simulink model "VEHICLE_DYN_TRAIN"  (R2019b)
settings: Solver=ode4  StartTime=0.0  StopTime=150  FixedStep=0.01  RelTol=1e-3
model workspace (MAT data in the model file):
  ACCEL = [0 0.000975932898663 -0.0414538855996 0.0440661905922 -0.0484817487001 0.0392964510644 -0.0693895143615 0.0261566921783 -0.0586295561215 0.0249771458914 -0.0595081132089 0.0233316013131 ... (544 elements, 17x32)]
  A_mc = 0.000491
  CMD_BR = [0 0 0 0 0 0 0 0 0 0 0 0 ... (15001 elements, 15001x1)]
  CMD_MODE = [1 1 1 1 1 1 1 1 1 1 1 1 ... (15001 elements, 15001x1)]
  CMD_ST = [0 0 0 0 0 0 0 0 0 0 0 0 ... (15001 elements, 15001x1)]
  CMD_T = [0 0.01 0.02 0.03 0.04 0.05 0.06 0.07 0.08 0.09 0.1 0.11 ... (2001 elements, 1x2001)]
  CMD_TH = [0 0 0 0 0 0 0 0 0 0 0 0 ... (15001 elements, 15001x1)]
  CMD_TM = [0 0.01 0.02 0.03 0.04 0.05 0.06 0.07 0.08 0.09 0.1 0.11 ... (15001 elements, 15001x1)]
  CMD_U = [10 10 10 10 10 10 10 10 10 10 10 10 ... (2001 elements, 1x2001)]
  CMD_UX = [0.1 0.1 0.1 0.1 0.1 0.1 0.1 0.1 0.1 0.1 0.1 0.1 ... (15001 elements, 15001x1)]
  COMMAND = [0  0  0  0  0  0; 0  0  0  0  -183.19381415  -6.40437742372; 0  0  0  0  1801.61134482  -6.40437742372; 0  0  0  0  -3911.54207947  -6.40437742372; 0  0  0  0  5117.32624779  -6.40437742372; 0  0  0  0  -8382.76633117  -6.40437742372; 0  0  0  0  5855.89111168  -6.40437742372; 0  0  0  0  2797.21692809  -6.40437742372; 0  0  0  0  -3762.9671569  -6.40437742372; 0  0  0  0  4210.58821039  -6.40437742372; 0  0  0  0  -2996.08013613  -6.40437742372; 0  0  0  0  5501.10926406  -6.40437742372; 0  0  0  0  1163.55068011  -6.40437742372; 0  0  0  0  -217.743214556  -6.40437742372; 0  0  0  0  2898.65655248  -6.40437742372; 0  0  0  0  2351.72581017  -6.40437742372; 0  0  0  0  936.262311224  -6.40437742372]
  C_q = 1.4e-06
  DATA_HMMWV.g = 9.81
  DATA_HMMWV.MU = 109.293567034
  DATA_HMMWV.MS = 2251.54374814
  DATA_HMMWV.VEHICLEMASS = 2688.71801627
  DATA_HMMWV.LA = 1.577476562
  DATA_HMMWV.LB = 1.724523438
  DATA_HMMWV.LC = 1.819402
  DATA_HMMWV.IXX = 1186.25695083
  DATA_HMMWV.IYY = 3535.89110102
  DATA_HMMWV.IZZ = 4110.07986387
  DATA_HMMWV.KS = [56433.9261732 56433.9261732 102219.884388 102219.884388]
  DATA_HMMWV.KT = [784944 784944 784944 784944]
  DATA_HMMWV.CS.RS = [-0.3391408 -0.332289470707 -0.325438141414 -0.318586812121 -0.311735482828 -0.304884153535 -0.298032824242 -0.291181494949 -0.284330165657 -0.277478836364 -0.270627507071 -0.263776177778 -0.256924848485 -0.250073519192 -0.243222189899 -0.236370860606 -0.229519531313 -0.22266820202 -0.215816872727 -0.208965543434 -0.202114214141 -0.195262884848 -0.188411555556 -0.181560226263 -0.17470889697 -0.167857567677 -0.161006238384 -0.154154909091 -0.147303579798 -0.140452250505 -0.133600921212 -0.126749591919 -0.119898262626 -0.113046933333 -0.10619560404 -0.0993442747475 -0.0924929454545 -0.0856416161616 -0.0787902868687 -0.0719389575758 -0.0650876282828 -0.0582362989899 -0.051384969697 -0.044533640404 -0.0376823111111 -0.0308309818182 -0.0239796525253 -0.0171283232323 -0.0102769939394 -0.00342566464646 0.00342566464646 0.0102769939394 0.0171283232323 0.0239796525253 0.0308309818182 0.0376823111111 0.044533640404 0.051384969697 0.0582362989899 0.0650876282828 0.0719389575758 0.0787902868687 0.0856416161616 0.0924929454545 0.0993442747475 0.10619560404 0.113046933333 0.119898262626 0.126749591919 0.133600921212 0.140452250505 0.147303579798 0.154154909091 0.161006238384 0.167857567677 0.17470889697 0.181560226263 0.188411555556 0.195262884848 0.202114214141 0.208965543434 0.215816872727 0.22266820202 0.229519531313 0.236370860606 0.243222189899 0.250073519192 0.256924848485 0.263776177778 0.270627507071 0.277478836364 0.284330165657 0.291181494949 0.298032824242 0.304884153535 0.311735482828 0.318586812121 0.325438141414 0.332289470707 0.3391408]
  DATA_HMMWV.CS.FDF = [-4248.0516471 -4239.67420418 -4225.63626971 -4206.16859138 -4181.50191691 -4151.866994 -4117.49457036 -4078.6153937 -4035.46021171 -3988.25977212 -3937.24482263 -3882.64611094 -3824.69438476 -3763.62039179 -3699.65487975 -3633.02859634 -3563.97228926 -3492.71670623 -3419.49259495 -3344.53070313 -3268.06177847 -3190.31656868 -3111.52582147 -3031.92028454 -2951.7307056 -2870.62252603 -2776.89068437 -2667.42140814 -2544.36901672 -2409.88782945 -2266.13216571 -2115.25634485 -1959.41468624 -1800.76150924 -1641.4511332 -1483.63787749 -1329.47606146 -1181.12000449 -1040.72402593 -910.442445139 -792.429581481 -688.738492968 -597.716409788 -515.80816219 -440.03739839 -367.427766603 -295.002915045 -219.786491931 -138.802145476 -49.0735238952 51.8288236509 162.22936071 281.055193785 407.628054481 541.269674406 681.301785165 827.046118366 977.824405614 1132.95837852 1295.36858067 1472.0381359 1661.32419521 1861.23445035 2069.77659305 2284.95831505 2504.78730808 2727.27126389 2950.4178742 3172.23483076 3390.7298253 3603.91054956 3809.78469528 4006.35995418 4191.64401802 4363.64457851 4524.5756402 4683.55471804 4840.88541831 4996.44105067 5150.09492481 5301.72035039 5451.1906371 5598.3790946 5743.15903257 5885.40376068 6024.98658862 6161.78082604 6295.65978264 6426.49676807 6554.16509202 6678.53806417 6799.48899417 6916.89119172 7030.61796648 7140.54262813 7246.53848634 7348.47885079 7446.23703115 7539.68633709 7628.7000783]
  DATA_HMMWV.CS.FDR = [-4359.2571876 -4354.21629512 -4343.74283127 -4328.06230688 -4307.40023276 -4281.98211973 -4252.03347861 -4217.7798202 -4179.44665534 -4137.25949483 -4091.4438495 -4042.22523015 -3989.82914761 -3934.4811127 -3876.40663622 -3815.831229 -3752.98040185 -3688.07966559 -3621.35453104 -3553.030509 -3483.33311031 -3412.48784578 -3340.72022622 -3268.25576245 -3195.31996528 -3121.7277695 -3038.93655817 -2944.39727451 -2839.35128227 -2725.03994522 -2602.70462711 -2473.58669171 -2338.92750277 -2199.96842406 -2057.95081932 -1914.11605233 -1769.70548684 -1625.96048661 -1484.1224154 -1345.43263697 -1211.13251508 -1082.42805518 -958.881518595 -838.498018865 -719.350253999 -599.510922001 -477.052720875 -350.048348627 -216.570503261 -74.6918827812 77.318355522 239.265853953 410.47181173 590.349120247 778.3106709 973.769355084 1176.13806419 1384.82968962 1599.25712277 1821.34171769 2055.89543661 2301.77114007 2557.5791448 2821.92976751 3093.43332495 3370.70013382 3652.34051085 3936.96477277 4223.18323631 4509.60621818 4794.8440351 5077.50700382 5356.20544104 5629.5496635 5896.14998792 6156.94821393 6416.88709644 6676.18645946 6934.83106248 7192.80566502 7450.09502655 7706.68390659 7962.55706462 8217.69926015 8472.09525268 8725.7298017 8978.58766672 9230.65360722 9481.91238271 9732.34875269 9981.94747665 10230.6933141 10478.5710245 10725.5653674 10971.6611023 11216.8429887 11461.095786 11704.4042538 11946.7531516 12188.1272388]
  DATA_HMMWV.CS.RS_INIT = -0.3391408
  DATA_HMMWV.CS.RS_SLOPE = 145.957077414
  DATA_HMMWV.AREA_FRONTAL = 3.58
  DATA_HMMWV.AIR_DENSITY = 1.22
  DATA_HMMWV.DRAG_COEFF = 0.7
  DATA_HMMWV.MAXPOWER = 225000
  DATA_HMMWV.IW = [40 40 40 40]
  DATA_HMMWV.RW = [0.548 0.548 0.548 0.548]
  DATA_HMMWV.HRCF = 0.85
  DATA_HMMWV.HRCR = 0.9
  DATA_HMMWV.HG = 0.9902452
  DATA_HMMWV.ZS_INIT = [0.9902452 0.9902452 0.9902452 0.9902452]
  DATA_HMMWV.XS_INIT = [-0.102204770695 -0.102204770695 -0.0516142786918 -0.0516142786918]
  DATA_HMMWV.XT_INIT = [-0.0087748080939 -0.0087748080939 -0.00802659668124 -0.00802659668124]
  DATA_HMMWV.ZT_INIT = [0.539225191906 0.539225191906 0.539973403319 0.539973403319]
  DATA_VESIM_CC_BRAKE.A_mc = 0.000491
  DATA_VESIM_CC_BRAKE.C_q = 1.4e-06
  DATA_VESIM_CC_BRAKE.F_cf = 80
  DATA_VESIM_CC_BRAKE.F_cs = 138
  DATA_VESIM_CC_BRAKE.F_z = -50097.6
  DATA_VESIM_CC_BRAKE.Gain_v = 70
  DATA_VESIM_CC_BRAKE.J_wheel = 32
  DATA_VESIM_CC_BRAKE.K_vb = 1500
  DATA_VESIM_CC_BRAKE.Kp_rpm = 2.7013
  DATA_VESIM_CC_BRAKE.Kp_v = 30
  DATA_VESIM_CC_BRAKE.L3 = 10
  DATA_VESIM_CC_BRAKE.MIN_TH = 0
  DATA_VESIM_CC_BRAKE.M_sprung = 4672
  DATA_VESIM_CC_BRAKE.M_unsprung = 220
  DATA_VESIM_CC_BRAKE.M_unsprung_front = 220
  DATA_VESIM_CC_BRAKE.M_vehicle = 5112
  DATA_VESIM_CC_BRAKE.N2 = 0
  DATA_VESIM_CC_BRAKE.N3 = 0.01
  DATA_VESIM_CC_BRAKE.P = 36
  DATA_VESIM_CC_BRAKE.P_0 = 10670
  DATA_VESIM_CC_BRAKE.P_gain = 0.0006
  DATA_VESIM_CC_BRAKE.R_wheel = 0.4412
  DATA_VESIM_CC_BRAKE.S_o = 3
  DATA_VESIM_CC_BRAKE.T2_r = 4
  DATA_VESIM_CC_BRAKE.Ti_rpm = 0.6464
  DATA_VESIM_CC_BRAKE.Ti_v = 2.5
  DATA_VESIM_CC_BRAKE.Tt_rpm = 0.0808
  DATA_VESIM_CC_BRAKE.Tt_v = 0.3125
  DATA_VESIM_CC_BRAKE.b = 170
  DATA_VESIM_CC_BRAKE.brake_Pw = [-3.96235801772; -3.96238075942; -0.895107722214; -0.895547395081; 35.9159438465; 72.7273668629; 152.485661058; 244.514654481; 330.408495385; 364.152342142; 462.316700341; 535.939857177; 618.766076338; 698.524620692; 775.215566044; 873.379969726; 950.0709454; 1029.82956556; 1106.52050333; 1174.00856829; 1241.49660293; 1339.66109; 1401.01384325; 1486.90776754; 1535.98996559; 1600.4103709; 1664.83081412; 1704.7101242; 1741.52177464; 1784.46875952; 1812.07749166; 1879.56559453; 1910.24195599; 1968.52709508; 2042.15044143; 2097.36794361; 2155.65309786; 2223.14114766; 2281.42629432; 2342.77908548]
  DATA_VESIM_CC_BRAKE.brake_V = [-1.14468402636e-08; 6.09303685082e-09; 2.9257815427e-07; 6.31682445149e-07; 8.18779962309e-07; 1.05849711081e-06; 1.41515318379e-06; 1.67826507702e-06; 1.8361367918e-06; 2.02323385108e-06; 2.22788040303e-06; 2.46760304614e-06; 2.60793442592e-06; 2.77165185063e-06; 2.90028906324e-06; 3.06985586096e-06; 3.17510657075e-06; 3.28035773841e-06; 3.41484157672e-06; 3.50255103574e-06; 3.61364699758e-06; 3.71890091255e-06; 3.82414933291e-06; 3.91770816494e-06; 4.00541487665e-06; 4.10481712919e-06; 4.17498625321e-06; 4.22761183705e-06; 4.29193021441e-06; 4.32116975331e-06; 4.3737935056e-06; 4.4322698361e-06; 4.49658729769e-06; 4.57844875735e-06; 4.67200575784e-06; 4.74802013391e-06; 4.81818834217e-06; 4.91759105259e-06; 4.99360588655e-06; 5.06962117839e-06]
  DATA_VESIM_CC_BRAKE.diff_efficiency = 0.94
  DATA_VESIM_CC_BRAKE.diff_wRatio = 6.052
  DATA_VESIM_CC_BRAKE.diff_w_ratio = 3.56
  DATA_VESIM_CC_BRAKE.engine_inertia = 0.53
  DATA_VESIM_CC_BRAKE.fmin_mg = [42.75 43.31 51.6 64.3 73.65 71.1 72.7 72.36]
  DATA_VESIM_CC_BRAKE.fmin_mg_na = [42.79 42.79 42.79 42.79 42.79 42.79 42.79 42.79]
  DATA_VESIM_CC_BRAKE.g = -9.8
  DATA_VESIM_CC_BRAKE.g_motor_eff = 1
  DATA_VESIM_CC_BRAKE.gr_motor = 0
  DATA_VESIM_CC_BRAKE.mdot_fuel = [5e-06 1e-05 2e-05 3e-05 4e-05 5e-05 6e-05 7e-05 8e-05]
  DATA_VESIM_CC_BRAKE.ms2mph = 2.23694
  DATA_VESIM_CC_BRAKE.n_tire = 4
  DATA_VESIM_CC_BRAKE.no_cyl = 8
  DATA_VESIM_CC_BRAKE.rpm0 = 83.7758040957
  DATA_VESIM_CC_BRAKE.rpm0_c = 1000
  DATA_VESIM_CC_BRAKE.rpm2rads = 0.10471975512
  DATA_VESIM_CC_BRAKE.rpm_e = [50 800 1000 1500 2000 2500 3000 3300]
  DATA_VESIM_CC_BRAKE.rpm_engine = [700 800 1000 1500 2000 2500 3000 3300]
  DATA_VESIM_CC_BRAKE.rpm_hi_idle = 3400
  DATA_VESIM_CC_BRAKE.rpm_idle = 750
  DATA_VESIM_CC_BRAKE.rpm_max_c = 3200
  DATA_VESIM_CC_BRAKE.rpm_rated = 3200
  DATA_VESIM_CC_BRAKE.torque_engine = [9.767  75.383  190.94  285.59  359.33  412.18  444.11  455.15  465.28; 15.303  80.318  196.25  293.4  371.76  431.33  472.12  494.11  497.32; 12.411  76.501  195.96  303.79  399.98  484.55  557.5  618.81  668.49; -4.524  61.314  188.26  308.88  423.2  531.2  632.9  728.28  817.34; -12.214  53.908  182.37  305.8  424.19  537.55  645.86  749.14  847.39; -35.77  30.439  158.78  281.67  399.12  511.13  617.7  718.82  814.5; -70  0  142.48  247.52  352.56  457.6  562.64  667.68  772.72; -75.889  -0.746  128.13  228.45  321.9  435.11  548.32  661.53  774.74]
  DATA_VESIM_CC_BRAKE.trq_scale = 0.46
  FORCE = [0 -4628.45620853 2357.84853747 -1841.82564621 -1727.75397473 1695.19792057 -1263.06335256 1524.31841051 -1649.98396845 -1537.1025145 -1335.96213703 1639.88309903 ... (493 elements, 17x29)]
  F_cf = 80
  F_cs = 138
  F_z = -50097.6
  Gain_v = 70
  J_wheel = 32
  K_vb = 1500
  Kp_rpm = 2.7013
  Kp_v = 30
  L3 = 10
  MIN_TH = 0
  M_sprung = 4672
  M_unsprung = 220
  M_unsprung_front = 220
  M_vehicle = 5112
  N2 = 0
  N3 = 0.01
  P = 36
  P_0 = 10670
  P_gain = 0.0006
  R_wheel = 0.4412
  SLIP = [0  0  0  0  0  0  0  0; -0.5  -0.5  -0.5  -0.5  -0.0351887274111  -0.0353738230462  -0.0256932606875  -0.025828461899; 0.5  0.5  0.5  0.5  0.935278264578  0.935683083202  0.934894152193  0.935259838194; -0.5  -0.5  -0.5  -0.5  -1.13059878896  -1.14410835605  -1.11878156022  -1.13275622068; -0.5  -0.5  -0.5  -0.5  1.27459495579  1.23136771502  1.24805246322  1.20169616214; 0.5  0.5  0.5  0.5  -1.39209196917  -1.31492534486  -1.36213294459  -1.27313134121; -0.5  -0.5  -0.5  -0.5  1.53834230958  1.52444006435  1.53915754649  1.52553193263; 0.5  -0.5  0.5  0.5  -1.53769354144  -1.55669825468  -1.53887189115  -1.55713779288; -0.5  -0.5  -0.5  -0.5  1.20354096649  1.12996957728  1.14188288665  1.05975342846; -0.5  0.5  -0.5  -0.5  -1.39844393881  -1.41657840122  -1.39247530022  -1.41016962351; -0.5  0.5  0.5  0.5  1.45508387354  1.20457176324  1.49318511219  1.31789576983; 0.5  0.5  -0.5  -0.5  -1.43949280681  -1.45477228425  -1.43518373844  -1.45165922694; -0.5  -0.5  -0.5  -0.409071280156  1.31587025686  1.35042722118  1.33080027133  1.36372378815; 0.5  0.5  0.5  0.5  -1.49514740357  -1.52618133061  -1.49024093571  -1.52178551982; -0.5  -0.5  -0.5  -0.5  0.548035911605  0.535056729347  0.504680092205  0.492118930826; 0.5  0.5  0.5  0.5  -1.44242137448  -1.56048589042  -1.46811475456  -1.56157095897; 0.5  0.5  0.5  -0.5  1.45666931557  1.52468060226  1.41014141796  1.50590281378]
  STATE = [0 4.33747954961e-06 -0.000147430460781 -3.72129119222e-05 -0.000284189368187 -0.000207128204422 -0.00055150808757 -0.000594561033148 -0.000967775941564 -0.00103412952076 -0.00143215770154 -0.00152470872631 ... (544 elements, 17x32)]
  STATES_INIT = [0 0 0.9902452 0 0 1.57079632679 0.01 0 0 0 0 0 0 0 0 0 -0.0087748080939 -0.0087748080939 -0.00802659668124 -0.00802659668124 -0.102204770695 -0.102204770695 -0.0516142786918 -0.0516142786918 0.0185451276203 0.0185451276203 0.0185194306581 0.0185194306581 0 0 0 0]
  SUSP = [0 -0.00875795294893 -0.00878173856984 -0.00830852863719 -0.00873591176348 -0.00870428588158 -0.00751721170558 -0.00851904716693 -0.00789923296531 -0.00838039895253 -0.00756270047902 -0.00866403364289 ... (612 elements, 17x36)]
  S_o = 3
  T2_r = 4
  TIRE = [0 0.0910654620457 -0.0936729683319 0.0717372732987 0.0513932148365 -0.0365035701266 -0.00739813929507 -0.0045484168787 0.0723881675257 0.0296400174207 -0.0169805208571 0.0207214713062 ... (408 elements, 17x24)]
  TIRELIFTOFF = [0; 0; 0; 0; 0; 0; 0; 0; 0; 0; 0; 0; 0; 0; 0; 0; 0]
  T_LENGTH = 2001
  T_STEP = 0.01
  T_STOP = 12.82
  T_TOTAL = 20
  Ti_rpm = 0.6464
  Ti_v = 2.5
  Tstop = [150 150 150 150 150 150 150 150 150 150 150 150 ... (15001 elements, 15001x1)]
  Tt_rpm = 0.0808
  Tt_v = 0.3125
  U_INIT = 0.01
  b = 170
  brake_Pw = [-3.96235801772; -3.96238075942; -0.895107722214; -0.895547395081; 35.9159438465; 72.7273668629; 152.485661058; 244.514654481; 330.408495385; 364.152342142; 462.316700341; 535.939857177; 618.766076338; 698.524620692; 775.215566044; 873.379969726; 950.0709454; 1029.82956556; 1106.52050333; 1174.00856829; 1241.49660293; 1339.66109; 1401.01384325; 1486.90776754; 1535.98996559; 1600.4103709; 1664.83081412; 1704.7101242; 1741.52177464; 1784.46875952; 1812.07749166; 1879.56559453; 1910.24195599; 1968.52709508; 2042.15044143; 2097.36794361; 2155.65309786; 2223.14114766; 2281.42629432; 2342.77908548]
  brake_V = [-1.14468402636e-08; 6.09303685082e-09; 2.9257815427e-07; 6.31682445149e-07; 8.18779962309e-07; 1.05849711081e-06; 1.41515318379e-06; 1.67826507702e-06; 1.8361367918e-06; 2.02323385108e-06; 2.22788040303e-06; 2.46760304614e-06; 2.60793442592e-06; 2.77165185063e-06; 2.90028906324e-06; 3.06985586096e-06; 3.17510657075e-06; 3.28035773841e-06; 3.41484157672e-06; 3.50255103574e-06; 3.61364699758e-06; 3.71890091255e-06; 3.82414933291e-06; 3.91770816494e-06; 4.00541487665e-06; 4.10481712919e-06; 4.17498625321e-06; 4.22761183705e-06; 4.29193021441e-06; 4.32116975331e-06; 4.3737935056e-06; 4.4322698361e-06; 4.49658729769e-06; 4.57844875735e-06; 4.67200575784e-06; 4.74802013391e-06; 4.81818834217e-06; 4.91759105259e-06; 4.99360588655e-06; 5.06962117839e-06]
  diff_efficiency = 0.94
  diff_wRatio = 6.052
  diff_w_ratio = 3.56
  end_time = 140
  engine_inertia = 0.53
  fmin_mg = [42.75 43.31 51.6 64.3 73.65 71.1 72.7 72.36]
  fmin_mg_na = [42.79 42.79 42.79 42.79 42.79 42.79 42.79 42.79]
  g = -9.8
  g_motor_eff = 1
  gr_motor = 0
  i = 5
  mdot_fuel = [5e-06 1e-05 2e-05 3e-05 4e-05 5e-05 6e-05 7e-05 8e-05]
  ms2mph = 2.23694
  n_tire = 4
  no_cyl = 8
  num_points = 14000
  num_points_fast = 140000
  rpm0 = 83.7758040957
  rpm0_c = 1000
  rpm2rads = 0.10471975512
  rpm_e = [50 800 1000 1500 2000 2500 3000 3300]
  rpm_engine = [700 800 1000 1500 2000 2500 3000 3300]
  rpm_hi_idle = 3400
  rpm_idle = 750
  rpm_max_c = 3200
  rpm_rated = 3200
  start_time = 0
  time_step = 0.01
  time_step_fast = 0.001
  torque_engine = [9.767  75.383  190.94  285.59  359.33  412.18  444.11  455.15  465.28; 15.303  80.318  196.25  293.4  371.76  431.33  472.12  494.11  497.32; 12.411  76.501  195.96  303.79  399.98  484.55  557.5  618.81  668.49; -4.524  61.314  188.26  308.88  423.2  531.2  632.9  728.28  817.34; -12.214  53.908  182.37  305.8  424.19  537.55  645.86  749.14  847.39; -35.77  30.439  158.78  281.67  399.12  511.13  617.7  718.82  814.5; -70  0  142.48  247.52  352.56  457.6  562.64  667.68  772.72; -75.889  -0.746  128.13  228.45  321.9  435.11  548.32  661.53  774.74]
  tout = [0; 0.01; 0.02; 0.03; 0.04; 0.05; 0.06; 0.07; 0.08; 0.09; 0.1; 0.11; 0.12; 0.13; 0.14; 0.15; 0.16]
  trq_scale = 0.46
values from neighbouring files (symbols this model uses):
  B = Ref(i:i+2,2)    [Calc_vref.m]    (also in Parameter_load.m = 0.1; VEHICLE_DYN_TRAIN_INIT.m = 0.25)
  Error_now = Error_now_array(end)    [RUN_SIMULATION_SHARED_NEW_POWERTRAIN.m]    (also in VEHICLE_DYN_TRAIN_INIT.m = 0)
  J = 0.075    [VEHICLE_DYN_TRAIN_INIT.m]
  K = 0.075    [VEHICLE_DYN_TRAIN_INIT.m]
  pid2tau_gain = 2.5    [VEHICLE_DYN_TRAIN_INIT.m]
  st_a_in = st_sc_out(end)    [RUN_SIMULATION_SHARED_NEW_POWERTRAIN.m]    (also in VEHICLE_DYN_TRAIN_INIT.m = 0)
  tau_a_in = tau_a_out(end)    [RUN_SIMULATION_SHARED_NEW_POWERTRAIN.m]    (also in VEHICLE_DYN_TRAIN_INIT.m = 0)
undefined symbols (not defined in the file or in its folder): adaptive_flag, autonomy_human_contain_gain, Bias_Distance, dt, error_lookuptable, human_autonomy_agreement_threshold, human_contain_min, human_response_dead_zone, human_torque_max, J_cal, kp_sc, model_lookuptable, Standard_Devices, steering_stable_threshold, UDP_Protocol, vdes, Xobs, Yobs
libraries: simulink x16, sldrtlib x3, dspstat3 x3, vrlib x2
(part 1 of 4)
settings Model: Creator=zhengys  LastModifiedBy=clicli
settings DataIOCC: LimitDataPoints=on  SaveFormat=Array  ReturnWorkspaceOutputs=off
settings OptimizationCC: BlockReduction=off  BooleanDataType=off  LifeSpan=inf
settings DebuggingCC: SaveWithParameterizedLinksMsg=none  UnderspecifiedInitializationDetection=Classic  MergeDetectMultiDrivingBlocksExec=none  SignalResolutionControl=TryResolveAllWithWarning  SFUnexpectedBacktrackingDiag=warning  SFNoUnconditionalDefaultTransitionDiag=warning  SFExecutionAtInitializationDiag=none  ArithmeticOperatorsInVariantConditions=warning
settings HardwareCC: ProdBitPerPointer=32  ProdBitPerSizeT=32  ProdBitPerPtrDiffT=32  ProdLargestAtomicFloat=None  ProdIntDivRoundTo=Undefined  ProdEndianess=Unspecified  ProdWordSize=32  ProdHWDeviceType=32-bit Generic  TargetUnknown=on
settings ModelReferenceCC: PropagateSignalLabelsOutOfModel=off
settings SFSimCC: SimUseLocalCustomCode=off  CustomCodeUndefinedFunction=UseInterfaceOnly
settings RTWCC: RTWUseLocalCustomCode=off
settings CodeAppCC: StateflowObjectComments=on
settings GRTTargetCC: TargetLangStandard=C89/C90 (ANSI)  GeneratePreprocessorConditionals=Disable all
settings ConfigComp: CovMetricSettings=dw  CovHtmlReporting=on  CovSaveCumulativeToWorkspaceVar=on  CovSaveSingleToWorkspaceVar=on  CovExternalEMLEnable=off  CovSFcnEnable=off

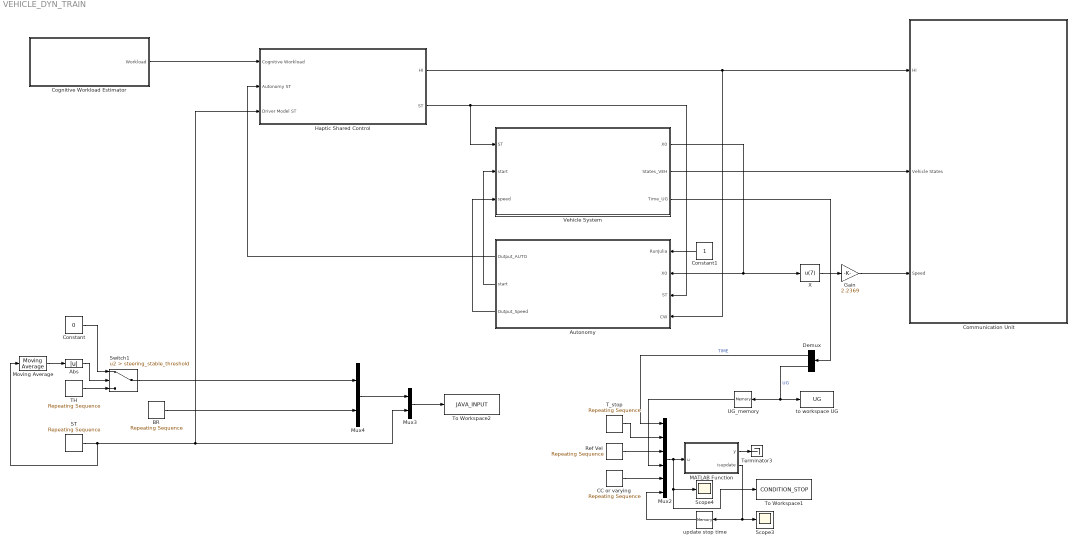
== system VEHICLE_DYN_TRAIN ==
  Abs : Abs
  Autonomy : Subsystem
  BR : simulink/Sources/Repeating Sequence  rep_seq_t=CMD_TM  rep_seq_y=CMD_BR
  CC or varying : simulink/Sources/Repeating Sequence  rep_seq_t=CMD_TM  rep_seq_y=CMD_MODE
  Cognitive Workload Estimator : Subsystem
  Communication Unit : Subsystem
  Constant : Constant  Value=0
  Constant1 : Constant
  Demux : Demux  Outputs=2
  Gain : Gain  Gain=2.2369
  Haptic Shared Control : Subsystem
  MATLAB Function : MATLAB Function  TreatAsAtomicUnit=on
  Moving Average : dspstat3/Moving Average  Method=Sliding window  ForgettingFactorPort=off  SpecifyWindowLength=on  WindowLength=50  ForgettingFactor=0.9  SimulateUsing=Code generation
  Mux2 : Mux  Inputs=6
  Mux3 : Mux  Inputs=2
  Mux4 : Mux  Inputs=2
  Ref Vel : simulink/Sources/Repeating Sequence  rep_seq_t=CMD_TM  rep_seq_y=CMD_UX
  ST : simulink/Sources/Repeating Sequence  rep_seq_t=CMD_TM  rep_seq_y=CMD_ST
  Scope3 : Scope
  Scope4 : Scope
  Switch1 : Switch  Criteria=u2 > Threshold  Threshold=steering_stable_threshold
  TH : simulink/Sources/Repeating Sequence  rep_seq_t=CMD_TM  rep_seq_y=CMD_TH
  T_stop : simulink/Sources/Repeating Sequence  rep_seq_t=CMD_TM  rep_seq_y=Tstop
  Terminator3 : Terminator
  To Workspace1 : ToWorkspace  VariableName=CONDITION_STOP  SampleTime=-1
  To Workspace2 : ToWorkspace  VariableName=JAVA_INPUT  SampleTime=-1
  UG_memory : Memory  InitialCondition=0.01
  Vehicle System : Subsystem
  X : Fcn  Expr=u(7)
  to workspace UG : ToWorkspace  VariableName=UG  SampleTime=-1
  update stop time : Memory
  wires:
  Mux4/1 -> Mux3/1
  ST/1 -> Haptic Shared Control/3(Driver Model ST), Mux3/2, Moving Average/1
  Mux3/1 -> To Workspace2/1
  Switch1/1 -> Mux4/1
  BR/1 -> Mux4/2
  TH/1 -> Switch1/3
  Constant/1 -> Switch1/1
  Moving Average/1 -> Abs/1
  Abs/1 -> Switch1/2
  Autonomy/2(start) -> Vehicle System/2(start)
  Gain/1 -> Communication Unit/3(Speed)
  Autonomy/1(Output_AUTO) -> Haptic Shared Control/2(Autonomy ST)
  Haptic Shared Control/2(ST) -> Vehicle System/1(ST), Autonomy/3(ST)
  Vehicle System/2(States_VEH) -> Communication Unit/2(Vehicle States)
  Autonomy/3(Output_Speed) -> Vehicle System/3(speed)
  Haptic Shared Control/1(HI) -> Autonomy/4(CW), Communication Unit/1(HI)
  Constant1/1 -> Autonomy/1(RunJulia)
  X/1 -> Gain/1
  Vehicle System/1(X0) -> Autonomy/2(X0), X/1
  MATLAB Function/1(y) -> Terminator3/1
  update stop time/1 -> Mux2/6
  MATLAB Function/2(isupdate) -> Scope3/1, update stop time/1
  Demux/2 -> UG_memory/1, to workspace UG/1  "UG"
  Mux2/1 -> To Workspace1/1, Scope4/1, MATLAB Function/1(u)
  UG_memory/1 -> Mux2/4
  T_stop/1 -> Mux2/2
  Vehicle System/3(Time_UG) -> Demux/1
  Demux/1 -> Mux2/1  "TIME"
  Ref Vel/1 -> Mux2/3
  CC or varying/1 -> Mux2/5
  Cognitive Workload Estimator/1(Workload) -> Haptic Shared Control/1(Cognitive Workload)
